simulink model "Grafica4"  (R2019a)
settings: Solver=VariableStepAuto  StartTime=0.0  StopTime=10.0  RelTol=1e-3
settings Model: Creator=rey_a  LastModifiedBy=rey_a

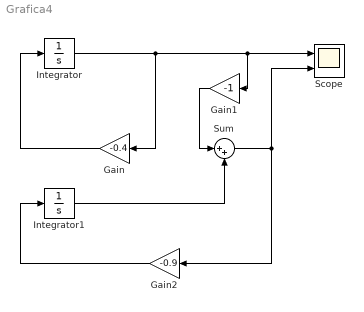
== system Grafica4 ==
  Gain : Gain  Gain=-0.4
  Gain1 : Gain  Gain=-1
  Gain2 : Gain  Gain=-0.9
  Integrator : Integrator  InitialCondition=800
  Integrator1 : Integrator
  Scope : Scope  NumInputPorts=2
  Sum : Sum  Inputs=|++
  wires:
  Gain/1 -> Integrator/1
  Integrator/1 -> Gain/1, Gain1/1, Scope/1
  Sum/1 -> Gain2/1, Scope/2
  Gain1/1 -> Sum/1
  Integrator1/1 -> Sum/2
  Gain2/1 -> Integrator1/1
